simulink model "asp1"  (R2016a)
settings: Solver=ode45  StartTime=0.0  StopTime=10.0  RelTol=1e-3
libraries: simulink x1
settings Model: Creator=Lugia  LastModifiedBy=17256
settings DataIOCC: LimitDataPoints=on  SaveFormat=Array
settings HardwareCC: ProdBitPerPointer=32  ProdLargestAtomicFloat=None  ProdIntDivRoundTo=Undefined  ProdEndianess=Unspecified  ProdWordSize=32  ProdHWDeviceType=32-bit Generic
settings ModelReferenceCC: PropagateSignalLabelsOutOfModel=off
settings ConfigComp: CovModelRefEnable=Off

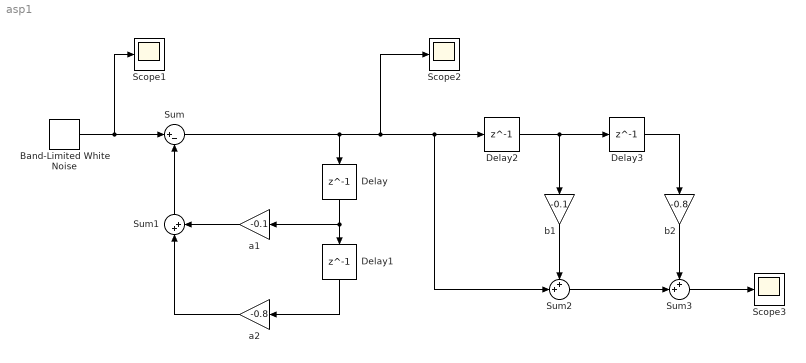
== system asp1 ==
  Band-Limited White Noise : simulink/Sources/Band-Limited White Noise  Cov=[0.1]  Ts=0.01  seed=[23341]
  Delay{,1..3} (4 alike) : Delay  DelayLength=1  InitialCondition=0
  Scope1 : Scope
  Scope2 : Scope
  Scope3 : Scope
  Sum : Sum  Inputs=|+-
  Sum1 : Sum  Inputs=|++
  Sum2 : Sum  Inputs=++|
  Sum3 : Sum  Inputs=++|
  a1 : Gain  Gain=-0.1
  a2 : Gain  Gain=-0.8
  b1 : Gain  Gain=-0.1
  b2 : Gain  Gain=-0.8
  wires:
  Band-Limited White Noise/1 -> Scope1/1, Sum/1
  Sum1/1 -> Sum/2
  Delay1/1 -> a2/1
  Delay/1 -> a1/1, Delay1/1
  a1/1 -> Sum1/2
  a2/1 -> Sum1/1
  Delay2/1 -> b1/1, Delay3/1
  Sum/1 -> Delay/1, Delay2/1, Sum2/2, Scope2/1
  Delay3/1 -> b2/1
  b1/1 -> Sum2/1
  b2/1 -> Sum3/1
  Sum2/1 -> Sum3/2
  Sum3/1 -> Scope3/1
